simulink subsystem "MG2Controller_HEVPowerSplit_refsub"  (R2023a)
settings: Solver=VariableStepAuto  StartTime=0.0  StopTime=10.0  RelTol=1e-3
undefined symbols (not defined in the file): hevcontrol
settings Model: Creator=isaacito  LastModifiedBy=isaacito
settings DebuggingCC: UnconnectedInputMsg=warning  UnconnectedOutputMsg=warning  UnconnectedLineMsg=warning
settings ModelReferenceCC: EnableRefExpFcnMdlSchedulingChecks=on
settings RTWCC: DLArmComputeVersion=19.05

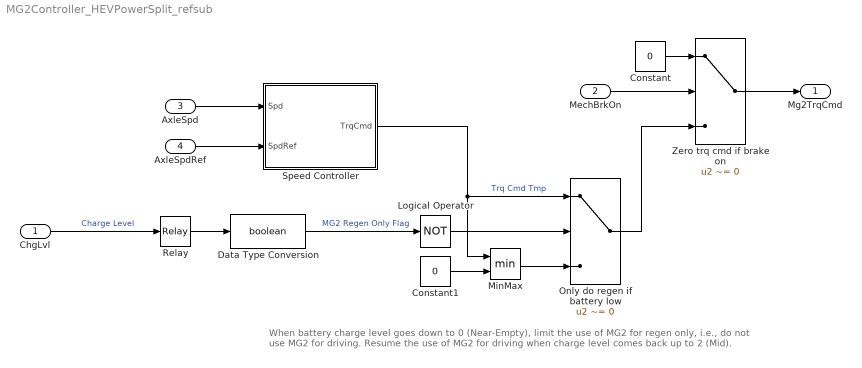
== system MG2Controller_HEVPowerSplit_refsub ==
  note: When battery charge level goes down to 0 (Near-Empty),
      | limit the use of MG2 for regen only, i.e., do not use MG2 for driving.
      | Resume the use of MG2 for driving when charge level comes back up to 2 (Mid).
  ChgLvl : Inport
  MechBrkOn : Inport  Port=2  OutDataTypeStr=boolean
      settings: AttributesFormatString=%<OutDataTypeStr>
  AxleSpd : Inport  Port=3  Unit=rpm
      settings: AttributesFormatString=%<Unit>
  AxleSpdRef : Inport  Port=4  Unit=rpm
      settings: AttributesFormatString=%<Unit>
  Constant : Constant  Value=0
  Constant1 : Constant  Value=0
  Data Type Conversion : DataTypeConversion  OutDataTypeStr=boolean  SaturateOnIntegerOverflow=off  RndMeth=Floor
  Logical Operator : Logic  Operator=NOT  AllPortsSameDT=off  OutDataTypeStr=boolean
  MinMax : MinMax  Inputs=2
  Only do regen if battery low : Switch  Criteria=u2 ~= 0  SaturateOnIntegerOverflow=off  InputSameDT=off
  Relay : Relay  OnSwitchValue=2  OffSwitchValue=0  OnOutputValue=0  OffOutputValue=1
  Speed Controller : Subsystem
      settings: PortSchema="{\"entries\":[{\"content\":{\"sides\":[{\"content\":{\"connectorIds\":[\"Out1\"]},\"type\":\"ConnectorPlacement.EquallySpacedRectSide\",\"uuid\":\"12b9f2c9-2b28-451b-ad36-7fe4150db485\"},{\"content\":{\"connectorIds\":[\"In1\",\"In2\"],\"side\":\"RIGHT\"},\"type\":\"ConnectorPlacement.EquallySpacedRectSide\",\"uuid\":\"c0fdf9a4-483a-4ddc-b663-6299fcc79327\"},{\"content\":{\"connectorIds\":[],\"side\":\"TOP\"},\"type\":\"ConnectorPlacement.EquallySpacedRectSide\",\"uuid\":\"3f20082e-8487-45e3-9fd7-d6d75741df4d\"}]},\"type\":\"ConnectorPlacement.EquallySpacedConnector\",\"uuid\":\"9361cdd3-74d8-46ee-ae7f-e2dde5d31ed1\"}],\"packageUris\":[\"http://schema.mathworks.com/mf0/Connector/R2020b\"],\"version\":\"1.0\"}"
  Zero trq cmd if brake on : Switch  Criteria=u2 ~= 0  SaturateOnIntegerOverflow=off  InputSameDT=off
  Mg2TrqCmd : Outport  Unit=N*m
      settings: AttributesFormatString=%<Unit>
  wires:
  Logical Operator/1 -> Only do regen if battery low/2
  AxleSpd/1 -> Speed Controller/1(Spd)
  Constant/1 -> Zero trq cmd if brake on/1
  MechBrkOn/1 -> Zero trq cmd if brake on/2
  AxleSpdRef/1 -> Speed Controller/2(SpdRef)
  Zero trq cmd if brake on/1 -> Mg2TrqCmd/1
  ChgLvl/1 -> Relay/1  "Charge Level"
  Only do regen if battery low/1 -> Zero trq cmd if brake on/3
  Constant1/1 -> MinMax/2
  Speed Controller/1(TrqCmd) -> MinMax/1, Only do regen if battery low/1  "Trq Cmd Tmp"
  Relay/1 -> Data Type Conversion/1
  MinMax/1 -> Only do regen if battery low/3
  Data Type Conversion/1 -> Logical Operator/1  "MG2 Regen Only Flag"

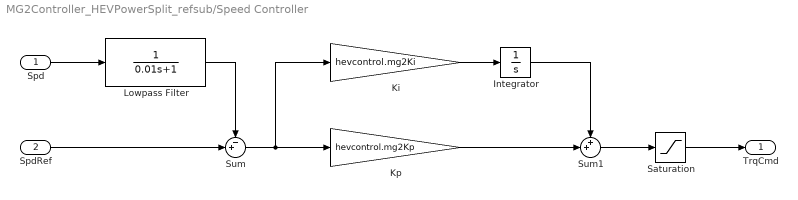
== system MG2Controller_HEVPowerSplit_refsub/Speed Controller ==
  Spd : Inport  Unit=rpm
      settings: AttributesFormatString=%<Unit>
  SpdRef : Inport  Port=2  Unit=rpm
      settings: AttributesFormatString=%<Unit>
  Integrator : Integrator  LimitOutput=on  UpperSaturationLimit=hevcontrol.mg2TrqMax_Nm  LowerSaturationLimit=-hevcontrol.mg2TrqMax_Nm
      settings: AttributesFormatString=|
      | %<UpperSaturationLimit>
      | %<LowerSaturationLimit>
  Ki : Gain  Gain=hevcontrol.mg2Ki
  Kp : Gain  Gain=hevcontrol.mg2Kp
  Lowpass Filter : TransferFcn  Denominator=[0.01 1]
  Saturation : Saturate  UpperLimit=hevcontrol.mg2TrqMax_Nm  LowerLimit=-hevcontrol.mg2TrqMax_Nm
      settings: AttributesFormatString=|
      | %<UpperLimit>
      | %<LowerLimit>
  Sum : Sum  Inputs=-+|
  Sum1 : Sum  Inputs=++|
  TrqCmd : Outport  Unit=N*m  VectorParamsAs1DForOutWhenUnconnected=off
      settings: AttributesFormatString=%<Unit>
  wires:
  Lowpass Filter/1 -> Sum/1
  Spd/1 -> Lowpass Filter/1
  Integrator/1 -> Sum1/1
  Kp/1 -> Sum1/2
  Ki/1 -> Integrator/1
  Sum/1 -> Ki/1, Kp/1
  Sum1/1 -> Saturation/1
  SpdRef/1 -> Sum/2
  Saturation/1 -> TrqCmd/1
